simulink model "sdl_testbed"  (R2022b)
settings: Solver=VariableStepAuto  StartTime=0.0  StopTime=5  RelTol=1e-3  AbsTol=1e-3  EnableMultiTasking=on
PreLoadFcn:
  | MFormulaCoeff.DryTarmac = [10 1.9 1 0.97];
  | MFormulaCoeff.WetTarmac = [12 2.3 0.82 1];
  | MFormulaCoeff.Snow         = [5 2 0.3 1];
  | MFormulaCoeff.Ice            = [4 2 0.1 1];
libraries: sdl_lib x22, nesl_utility x9, fl_ps_legacy_lib x5, fl_lib x4, simulink x1
(part 3 of 3)

== system sdl_testbed/Center Differential/Lockup/Lag ==
  PS Gain : fl_ps_legacy_lib/Legacy Physical Signals/Functions/PS Gain  gain=1/0.01
  PS Integrator : fl_ps_legacy_lib/Legacy Physical Signals/Linear Operators/PS Integrator  x0=0
      settings: InternalSimscapePortConfiguration="{\"Bottom\":[],\"Left\":[{\"id\":\"I\",\"label\":\"\",\"type\":\"input\"}],\"Right\":[{\"id\":\"O\",\"label\":\"\",\"type\":\"output\"}],\"Top\":[]}"
  PS Subtract : fl_ps_legacy_lib/Legacy Physical Signals/Functions/PS Subtract
  I : PMIOPort  Side=Left
  O : PMIOPort  Port=2  Side=Right
  connections:
  PS Subtract/LConn2 -- PS Gain/RConn1 -- O/RConn1
  I/RConn1 -- PS Subtract/LConn1
  PS Gain/LConn1 -- PS Integrator/RConn1
  PS Integrator/LConn1 -- PS Subtract/RConn1

== system sdl_testbed/Road/Select MF Coefficients/Filter MF Coeff LF ==
  In : Inport
  Gain : Gain  Gain=1/b
  Integrator : Integrator  InitialCondition=x_initial*b
  Sum : Sum  Inputs=|+-  InputSameDT=on  SaturateOnIntegerOverflow=on  OutDataTypeStr=Inherit: Same as first input
  Out : Outport  VectorParamsAs1DForOutWhenUnconnected=off
  wires:
  Sum/1 -> Integrator/1
  In/1 -> Sum/1
  Integrator/1 -> Gain/1
  Gain/1 -> Sum/2, Out/1

== system sdl_testbed/Road/Select MF Coefficients/Filter MF Coeff LR ==
  In : Inport
  Gain : Gain  Gain=1/b
  Integrator : Integrator  InitialCondition=x_initial*b
  Sum : Sum  Inputs=|+-  InputSameDT=on  SaturateOnIntegerOverflow=on  OutDataTypeStr=Inherit: Same as first input
  Out : Outport  VectorParamsAs1DForOutWhenUnconnected=off
  wires:
  Sum/1 -> Integrator/1
  In/1 -> Sum/1
  Integrator/1 -> Gain/1
  Gain/1 -> Sum/2, Out/1

== system sdl_testbed/Road/Select MF Coefficients/Filter MF Coeff RF ==
  In : Inport
  Gain : Gain  Gain=1/b
  Integrator : Integrator  InitialCondition=x_initial*b
  Sum : Sum  Inputs=|+-  InputSameDT=on  SaturateOnIntegerOverflow=on  OutDataTypeStr=Inherit: Same as first input
  Out : Outport  VectorParamsAs1DForOutWhenUnconnected=off
  wires:
  Gain/1 -> Out/1, Sum/2
  Integrator/1 -> Gain/1
  In/1 -> Sum/1
  Sum/1 -> Integrator/1

== system sdl_testbed/Road/Select MF Coefficients/Filter MF Coeff RR ==
  In : Inport
  Gain : Gain  Gain=1/b
  Integrator : Integrator  InitialCondition=x_initial*b
  Sum : Sum  Inputs=|+-  InputSameDT=on  SaturateOnIntegerOverflow=on  OutDataTypeStr=Inherit: Same as first input
  Out : Outport  VectorParamsAs1DForOutWhenUnconnected=off
  wires:
  Gain/1 -> Out/1, Sum/2
  Integrator/1 -> Gain/1
  In/1 -> Sum/1
  Sum/1 -> Integrator/1

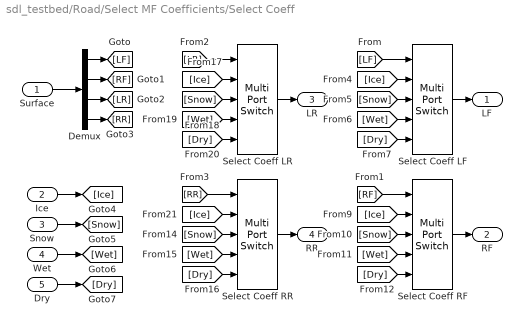
== system sdl_testbed/Road/Select MF Coefficients/Select Coeff ==
  Surface : Inport
  Ice : Inport  Port=2
  Snow : Inport  Port=3
  Wet : Inport  Port=4
  Dry : Inport  Port=5
  Demux : Demux
  Select Coeff LF : MultiPortSwitch  Inputs=4  SaturateOnIntegerOverflow=off  InputSameDT=off
  Select Coeff LR : MultiPortSwitch  Inputs=4  SaturateOnIntegerOverflow=off  InputSameDT=off
  Select Coeff RF : MultiPortSwitch  Inputs=4  SaturateOnIntegerOverflow=off  InputSameDT=off
  Select Coeff RR : MultiPortSwitch  Inputs=4  SaturateOnIntegerOverflow=off  InputSameDT=off
  LF : Outport  VectorParamsAs1DForOutWhenUnconnected=off
  RF : Outport  Port=2  VectorParamsAs1DForOutWhenUnconnected=off
  LR : Outport  Port=3  VectorParamsAs1DForOutWhenUnconnected=off
  RR : Outport  Port=4  VectorParamsAs1DForOutWhenUnconnected=off
  wires:
  Wet/1 -> [Wet]
  Surface/1 -> Demux/1
  Ice/1 -> [Ice]
  Snow/1 -> [Snow]
  Dry/1 -> [Dry]
  Select Coeff LF/1 -> LF/1
  Demux/1 -> [LF]
  Demux/2 -> [RF]
  Demux/3 -> [LR]
  Demux/4 -> [RR]
  [LF] -> Select Coeff LF/1
  [Ice] -> Select Coeff LF/2
  [Snow] -> Select Coeff LF/3
  [Wet] -> Select Coeff LF/4
  [Dry] -> Select Coeff LF/5
  Select Coeff RF/1 -> RF/1
  [RF] -> Select Coeff RF/1
  [Ice] -> Select Coeff RF/2
  [Snow] -> Select Coeff RF/3
  [Wet] -> Select Coeff RF/4
  [Dry] -> Select Coeff RF/5
  Select Coeff LR/1 -> LR/1
  [LR] -> Select Coeff LR/1
  [Ice] -> Select Coeff LR/2
  [Snow] -> Select Coeff LR/3
  [Wet] -> Select Coeff LR/4
  [Dry] -> Select Coeff LR/5
  Select Coeff RR/1 -> RR/1
  [RR] -> Select Coeff RR/1
  [Ice] -> Select Coeff RR/2
  [Snow] -> Select Coeff RR/3
  [Wet] -> Select Coeff RR/4
  [Dry] -> Select Coeff RR/5
